simulink model "buoy"  (R2025a)
settings: Solver=FixedStepAuto  StartTime=0.0  StopTime=10.0  FixedStep=5e-5  RelTol=1e-3
libraries: spsVoltageMeasurementLib x5, spsSeriesRLCBranchLib x3, spsBuckConverterLib x1, spsGroundLib x1, spsPermanentMagnetSynchronousMachineLib x1, spsUniversalBridgeLib x1, sps_lib x1
settings Model: Creator=jacks  LastModifiedBy=jacks
settings SolverCC: ZeroCrossAlgorithm=Adaptive

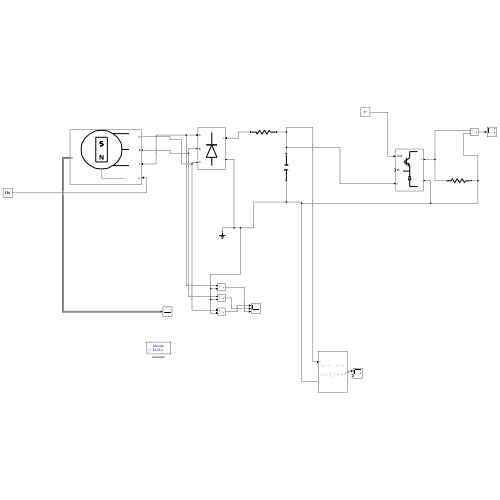
[thumbnail: Simulink's stored preview of the top-level diagram]
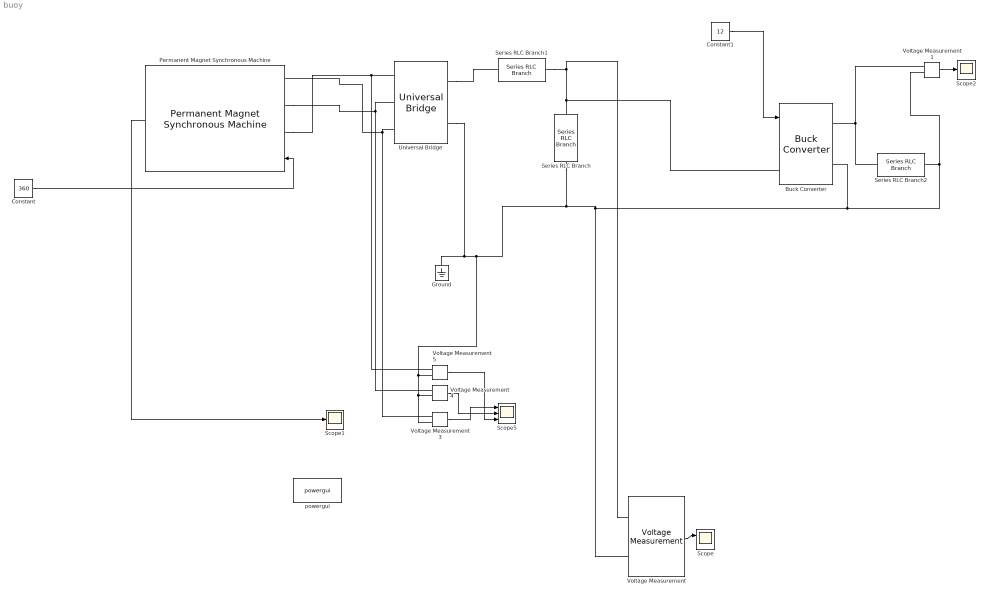
== system buoy ==
  Buck Converter : spsBuckConverterLib/Buck Converter  ModelType=Average model (No rectifier mode)  Ron=1e-3  Rs=1e6  Cs=inf  Vforward=[0,0]  Ron_Diode=1e-3  Rs_Diode=1e6  Cs_Diode=inf  Vf_Diode=1e-3  Rs_CurrentSource=inf  Ron_ACsource=1e-3
      settings: LibrarySourceBlock=sps_lib/Power Electronics/Buck Converter
  Constant : Constant  Value=360
  Constant1 : Constant  Value=12
  Ground : spsGroundLib/Ground  LConnTagsString=a
  Permanent Magnet Synchronous Machine : spsPermanentMagnetSynchronousMachineLib/Permanent Magnet Synchronous Machine  NbPhases=3  FluxDistribution=Sinusoidal  RotorType=Round  MechanicalLoad=Speed w  PresetModel=No  ShowDetailedParameters=on  MeasurementBus=on  Resistance=0.144  Inductance=8.5e-3  dqInductances=[8.5e-3,8.5e-3]  La=0.0001395  MachineConstant=Torque Constant (N.m / A_peak)  Flux=0.0025  VoltageCst=6.3483  TorqueCst=0.0525  Flat=120  Mechanical=[08.35e-5 1e-4 7 0]  PolePairs=14  InitialConditions=[0,0, 0,0]  InitialConditions5ph=[0 0 0 0 0 0]  RefAngle=90 degrees behind phase A axis (modified Park)  IterativeDiscreteModel=Trapezoidal non iterative  TsBlock=-1  TsPowergui=0
  Scope : Scope  NumInputPorts=2
      settings: ActiveDisplayYMinimum=0.55100123687361346  ActiveDisplayYMaximum=35.84151367121855
  Scope1 : Scope
      settings: ActiveDisplayYMinimum=-0.28592697422417546  ActiveDisplayYMaximum=1.1933882340446553
  Scope2 : Scope
      settings: ActiveDisplayYMinimum=-6.88626800051231E+305  ActiveDisplayYMaximum=1.801837262823849E+307  DataLoggingVariableName=ScopeData2
  Scope5 : Scope  NumInputPorts=3
      settings: ActiveDisplayYMinimum=-48.826027188456806  ActiveDisplayYMaximum=47.147776815060368  DataLoggingVariableName=ScopeData5
  Series RLC Branch : spsSeriesRLCBranchLib/Series RLC Branch  LConnTagsString=__new0  RConnTagsString=__new0  BranchType=C  Resistance=1  Inductance=1e-3  SetiL0=off  InitialCurrent=0  Capacitance=0.0047  Setx0=off  InitialVoltage=0  Measurements=Branch voltage and current
  Series RLC Branch1 : spsSeriesRLCBranchLib/Series RLC Branch  LConnTagsString=__new0  RConnTagsString=__new0  BranchType=R  Resistance=0.5  Inductance=1e-3  SetiL0=off  InitialCurrent=0  Capacitance=0.0047  Setx0=off  InitialVoltage=0  Measurements=Branch voltage and current
  Series RLC Branch2 : spsSeriesRLCBranchLib/Series RLC Branch  LConnTagsString=__new0  RConnTagsString=__new0  BranchType=R  Resistance=100  Inductance=1e-3  SetiL0=off  InitialCurrent=0  Capacitance=1e-6  Setx0=off  InitialVoltage=0  Measurements=None
  Universal Bridge : spsUniversalBridgeLib/Universal Bridge  Arms=3  SnubberResistance=1e5  SnubberCapacitance=inf  Device=Diodes  Ron=1e-3  Lon=0  ForwardVoltages="[  0  0  ]"  ForwardVoltage=0  GTOparameters=[ 10e-6 , 20e-6 ]  IGBTparameters=[ 1e-6 , 2e-6 ]  Measurements=UAB UBC UCA UDC voltages  Measurements_2=None  converterType=Rectifier
  Voltage Measurement{,1,3..5} (5 alike) : spsVoltageMeasurementLib/Voltage Measurement  PhasorSimulation=off  OutputType=Complex  PSBequivalent=0
  powergui : sps_lib/powergui  Priority=1  SimulationMode=Discrete  SampleTime=5e-5  frequency=60  Iterations=50  frequencyindice=0  Pbase=100e6  ErrMax=1e-4  UnitsV=kV  UnitsW=MW  buscounter=0  FunctionMessages=off  echomessages=off  EnableUseOfTLC=off  CurrentSourceSwitches=off  DisableSnubberDevices=off  DisableRonSwitches=off  DisableVfSwitches=off  DisplayEquations=off  AutomaticDiscreteSolvers=on  SolverType=Tustin/Backward Euler (TBE)  Interpol=off  ExternalGateDelay=off  methode=off  Ts=100  x0status=blocks  SPID=on  SwTol=0  HookPort=off  NonlinearTolerance=1e-4  nMaxIteration=100  ContinueOnMaxIteration=off  RestoreLinks=warning  ResistiveCurrentMeasurement=off  Frange=[0:2:500]  Ylog=off  Xlog=on  ShowGrid=off  save=off  variable=ZData  structure=0  ZoomFFT=off  StartTime=0.0  cycles=1  DisplayStyle=1  fundamental=60  FreqAxis=off  MaxFrequency=1000  frequencyindicesteady=1  RmsSteady=1  display=off
  wires:
  Voltage Measurement/1 -> Scope/1
  Constant/1 -> Permanent Magnet Synchronous Machine/1
  Permanent Magnet Synchronous Machine/1 -> Scope1/1
  Voltage Measurement3/1 -> Scope5/1
  Voltage Measurement4/1 -> Scope5/2
  Voltage Measurement5/1 -> Scope5/3
  Constant1/1 -> Buck Converter/1
  Voltage Measurement1/1 -> Scope2/1
  connections:
  Voltage Measurement5/LConn2 -- Voltage Measurement4/LConn2 -- Voltage Measurement3/LConn2 -- Ground/LConn1 -- Universal Bridge/RConn2 -- Series RLC Branch/RConn1 -- Voltage Measurement1/LConn2 -- Series RLC Branch2/RConn1 -- Buck Converter/RConn2 -- Voltage Measurement/LConn2
  Series RLC Branch/LConn1 -- Voltage Measurement/LConn1 -- Series RLC Branch1/LConn1 -- Buck Converter/LConn1
  Permanent Magnet Synchronous Machine/LConn1 -- Voltage Measurement5/LConn1 -- Universal Bridge/LConn1
  Universal Bridge/RConn1 -- Series RLC Branch1/RConn1
  Permanent Magnet Synchronous Machine/LConn2 -- Voltage Measurement4/LConn1 -- Universal Bridge/LConn2
  Universal Bridge/LConn3 -- Voltage Measurement3/LConn1 -- Permanent Magnet Synchronous Machine/LConn3
  Series RLC Branch2/LConn1 -- Voltage Measurement1/LConn1 -- Buck Converter/RConn1
